simulink model "frameBasedSobelFilter"  (R2023a)
settings: Solver=FixedStepDiscrete  StartTime=0.0  StopTime=2  RelTol=1e-3
values from neighbouring files (symbols this model uses):
  c = 752    [setupFrame.m]
  r = 480    [setupFrame.m]
libraries: hdlsllib x16, visionsources x1
Description:
  | Sobel Edge Detection Using the MATLAB(R) Function Block
  | This example shows how to use HDL Coder(TM) to check,
  | generate, and verify HDL code for a Sobel Edge Detection
  | block built using the MATLAB Function block.
settings Model: Creator=The MathWorks, Inc.  LastModifiedBy=dskap
settings SolverCC: AlgebraicLoopSolver=TrustRegion
settings DataIOCC: LimitDataPoints=on  SaveFormat=Array  SignalLogging=off  ReturnWorkspaceOutputs=off
settings OptimizationCC: BlockReduction=off  ConditionallyExecuteInputs=off  DefaultParameterBehavior=Inlined  ExpressionDepthLimit=2147483647  InitFltsAndDblsToZero=on  EfficientMapNaN2IntZero=off  LifeSpan=inf
settings DebuggingCC: AlgebraicLoopMsg=error  SaveWithParameterizedLinksMsg=none  UnderspecifiedInitializationDetection=Classic  MergeDetectMultiDrivingBlocksExec=none  SignalResolutionControl=TryResolveAllWithWarning  MultiTaskDSMMsg=warning  MultiTaskCondExecSysMsg=none  SingleTaskRateTransMsg=error  IntegerOverflowMsg=none  ParameterPrecisionLossMsg=none  FcnCallInpInsideContextMsg=warning  UnconnectedInputMsg=warning  UnconnectedOutputMsg=warning  UnconnectedLineMsg=warning  AllowSymbolicDim=off  StateNameClashWarn=warning  StrictBusMsg=ErrorOnBusTreatedAsVector  SFUnexpectedBacktrackingDiag=warning  SFNoUnconditionalDefaultTransitionDiag=warning  SFExecutionAtInitializationDiag=none  IntegerSaturationMsg=none  ArithmeticOperatorsInVariantConditions=warning
settings HardwareCC: ProdBitPerPointer=32  ProdBitPerSizeT=32  ProdBitPerPtrDiffT=32  ProdLargestAtomicFloat=None  ProdIntDivRoundTo=Undefined  ProdEndianess=Unspecified  ProdWordSize=32  ProdHWDeviceType=ASIC/FPGA  TargetHWDeviceType=32-bit Generic  ProdEqTarget=off
settings ModelReferenceCC: EnableRefExpFcnMdlSchedulingChecks=on  PropagateSignalLabelsOutOfModel=off
settings SFSimCC: SimUseLocalCustomCode=off  CustomCodeUndefinedFunction=UseInterfaceOnly
settings RTWCC: RTWUseLocalCustomCode=off  DLArmComputeVersion=19.05
settings CodeAppCC: StateflowObjectComments=on
settings GRTTargetCC: TargetFcnLib=ansi_tfl_tmw.mat  TargetLangStandard=C89/C90 (ANSI)  CombineOutputUpdateFcns=off  GRTInterface=on
settings ConfigComp: CovMetricSettings=dw  CovSaveCumulativeToWorkspaceVar=on  CovSaveSingleToWorkspaceVar=on  CovExternalEMLEnable=off

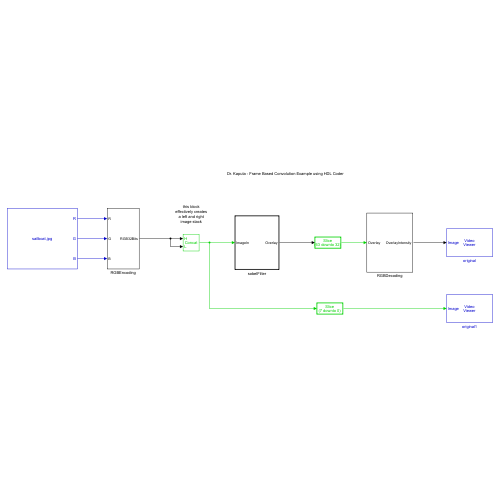
[thumbnail: Simulink's stored preview of the top-level diagram]
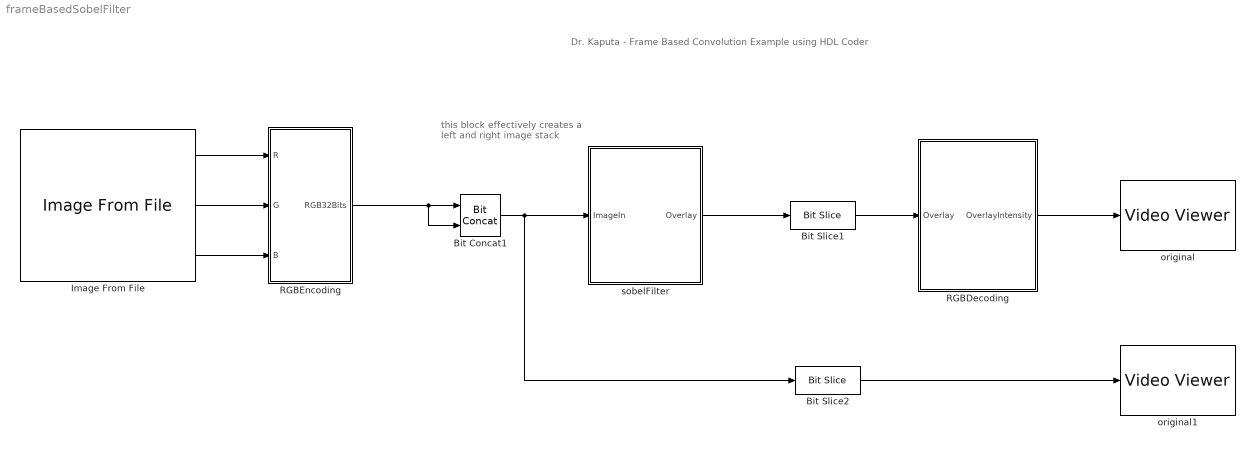
== system frameBasedSobelFilter ==
  note: this block effectively creates a left and right image stack
  note: Dr. Kaputa - Frame Based Convolution Example using HDL Coder
  Bit Concat1 : hdlsllib/Logic and Bit Operations/Bit Concat  numInputs=2
  Bit Slice1 : hdlsllib/Logic and Bit Operations/Bit Slice  lidx=63  ridx=32
  Bit Slice2 : hdlsllib/Logic and Bit Operations/Bit Slice  lidx=7  ridx=0
  Image From File : visionsources/Image From File  Tag=vipblks_nd  FileName=sailboat.jpg  Ts=1  imagePorts=Separate color signals  OutPortLabels=R|G|B  ImageDataType=Inherit from input image  sdImageDataType=uint(8)  Signed=on  WordLength=16  FractionLengthMode=User-defined  FractionLength=15
  RGBDecoding : Subsystem
  RGBEncoding : Subsystem
  original : VideoViewer  FigPos=[-1279 718 1280 622.666666666667]
  original1 : VideoViewer  FigPos=[-1279 718 1280 622.666666666667]
  sobelFilter : Subsystem  TreatAsAtomicUnit=on
  wires:
  sobelFilter/1(Overlay) -> Bit Slice1/1
  Image From File/1 -> RGBEncoding/1(R)
  Image From File/2 -> RGBEncoding/2(G)
  Image From File/3 -> RGBEncoding/3(B)
  RGBEncoding/1(RGB32Bits) -> Bit Concat1/2, Bit Concat1/1
  Bit Concat1/1 -> Bit Slice2/1, sobelFilter/1(ImageIn)
  RGBDecoding/1(OverlayIntensity) -> original/1
  Bit Slice1/1 -> RGBDecoding/1(Overlay)
  Bit Slice2/1 -> original1/1

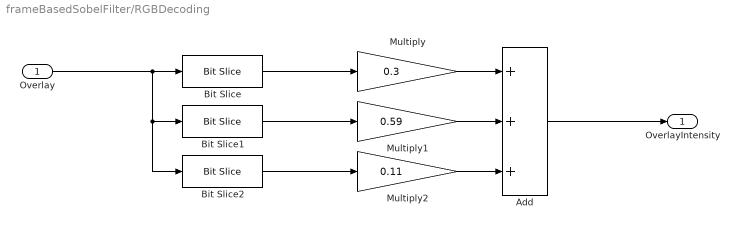
== system frameBasedSobelFilter/RGBDecoding ==
  Overlay : Inport
  Add : Sum  Inputs=+++  OutDataTypeStr=uint8
  Bit Slice : hdlsllib/Logic and Bit Operations/Bit Slice  lidx=23  ridx=16
  Bit Slice1 : hdlsllib/Logic and Bit Operations/Bit Slice  lidx=15  ridx=8
  Bit Slice2 : hdlsllib/Logic and Bit Operations/Bit Slice  lidx=7  ridx=0
  Multiply : Gain  Gain=0.3  OutDataTypeStr=uint8
  Multiply1 : Gain  Gain=0.59  OutDataTypeStr=uint8
  Multiply2 : Gain  Gain=0.11  OutDataTypeStr=uint8
  OverlayIntensity : Outport
  wires:
  Multiply/1 -> Add/1
  Overlay/1 -> Bit Slice2/1, Bit Slice1/1, Bit Slice/1
  Bit Slice/1 -> Multiply/1
  Bit Slice2/1 -> Multiply2/1
  Add/1 -> OverlayIntensity/1
  Bit Slice1/1 -> Multiply1/1
  Multiply2/1 -> Add/3
  Multiply1/1 -> Add/2

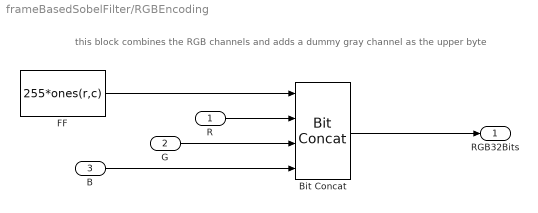
== system frameBasedSobelFilter/RGBEncoding ==
  note: this block combines the RGB channels and adds a dummy gray channel as the upper byte
  R : Inport
  G : Inport  Port=2
  B : Inport  Port=3
  Bit Concat : hdlsllib/Logic and Bit Operations/Bit Concat  numInputs=4
  FF : Constant  Value=255*ones(r,c)  OutDataTypeStr=uint8  SampleTime=1
  RGB32Bits : Outport
  wires:
  FF/1 -> Bit Concat/1
  Bit Concat/1 -> RGB32Bits/1
  R/1 -> Bit Concat/2
  G/1 -> Bit Concat/3
  B/1 -> Bit Concat/4

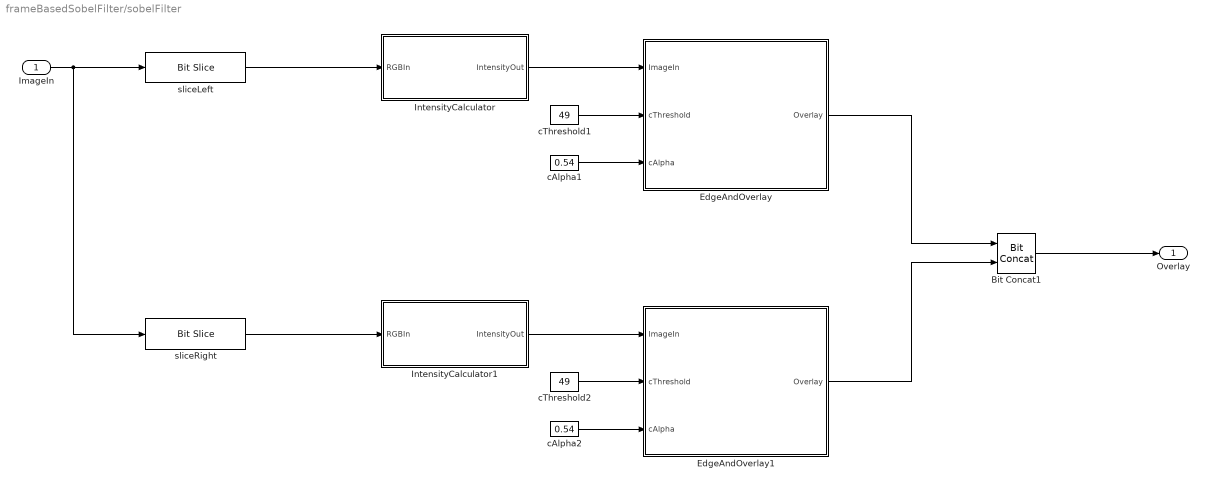
== system frameBasedSobelFilter/sobelFilter ==
  ImageIn : Inport
  Bit Concat1 : hdlsllib/Logic and Bit Operations/Bit Concat  numInputs=2
  EdgeAndOverlay : MATLAB Function  TreatAsAtomicUnit=on
  EdgeAndOverlay1 : MATLAB Function  TreatAsAtomicUnit=on
  IntensityCalculator : Subsystem
  IntensityCalculator1 : Subsystem
  cAlpha1 : Constant  Value=0.54  OutDataTypeStr=fixdt(0,16,15)  SampleTime=1
  cAlpha2 : Constant  Value=0.54  OutDataTypeStr=fixdt(0,16,15)  SampleTime=1
  cThreshold1 : Constant  Value=49  OutDataTypeStr=uint8  SampleTime=1
  cThreshold2 : Constant  Value=49  OutDataTypeStr=uint8  SampleTime=1
  sliceLeft : hdlsllib/Logic and Bit Operations/Bit Slice  lidx=63  ridx=32
  sliceRight : hdlsllib/Logic and Bit Operations/Bit Slice  lidx=31  ridx=0
  Overlay : Outport
  wires:
  cThreshold1/1 -> EdgeAndOverlay/2(cThreshold)
  cAlpha1/1 -> EdgeAndOverlay/3(cAlpha)
  IntensityCalculator/1(IntensityOut) -> EdgeAndOverlay/1(ImageIn)
  sliceLeft/1 -> IntensityCalculator/1(RGBIn)
  ImageIn/1 -> sliceLeft/1, sliceRight/1
  sliceRight/1 -> IntensityCalculator1/1(RGBIn)
  IntensityCalculator1/1(IntensityOut) -> EdgeAndOverlay1/1(ImageIn)
  cAlpha2/1 -> EdgeAndOverlay1/3(cAlpha)
  EdgeAndOverlay1/1(Overlay) -> Bit Concat1/2
  cThreshold2/1 -> EdgeAndOverlay1/2(cThreshold)
  Bit Concat1/1 -> Overlay/1
  EdgeAndOverlay/1(Overlay) -> Bit Concat1/1

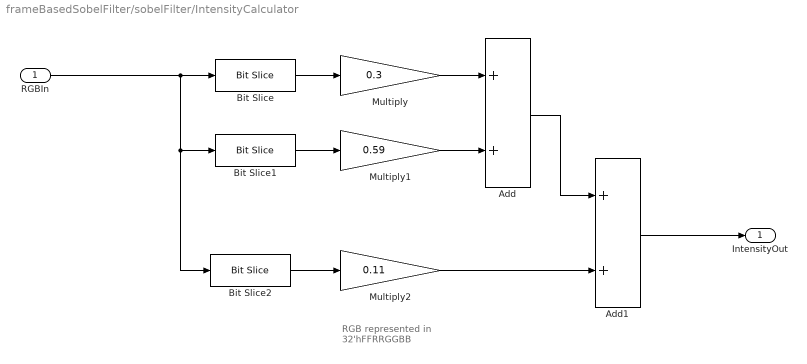
== system frameBasedSobelFilter/sobelFilter/IntensityCalculator ==
  note: RGB represented in
      | 32'hFFRRGGBB
  RGBIn : Inport
  Add : Sum  OutDataTypeStr=uint8
  Add1 : Sum  OutDataTypeStr=uint8
  Bit Slice : hdlsllib/Logic and Bit Operations/Bit Slice  lidx=23  ridx=16
  Bit Slice1 : hdlsllib/Logic and Bit Operations/Bit Slice  lidx=15  ridx=8
  Bit Slice2 : hdlsllib/Logic and Bit Operations/Bit Slice  lidx=7  ridx=0
  Multiply : Gain  Gain=0.3  OutDataTypeStr=uint8
  Multiply1 : Gain  Gain=0.59  OutDataTypeStr=uint8
  Multiply2 : Gain  Gain=0.11  OutDataTypeStr=uint8
  IntensityOut : Outport
  wires:
  Bit Slice1/1 -> Multiply1/1
  Multiply2/1 -> Add1/2
  Multiply/1 -> Add/1
  Multiply1/1 -> Add/2
  Bit Slice/1 -> Multiply/1
  Add/1 -> Add1/1
  RGBIn/1 -> Bit Slice2/1, Bit Slice1/1, Bit Slice/1
  Add1/1 -> IntensityOut/1
  Bit Slice2/1 -> Multiply2/1

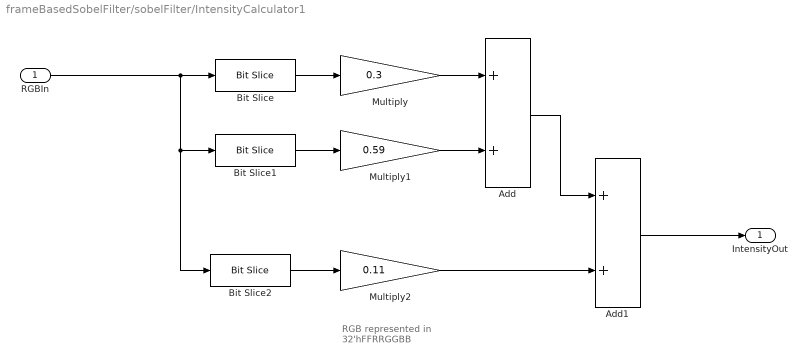
== system frameBasedSobelFilter/sobelFilter/IntensityCalculator1 ==
  note: RGB represented in
      | 32'hFFRRGGBB
  RGBIn : Inport
  Add : Sum  OutDataTypeStr=uint8
  Add1 : Sum  OutDataTypeStr=uint8
  Bit Slice : hdlsllib/Logic and Bit Operations/Bit Slice  lidx=23  ridx=16
  Bit Slice1 : hdlsllib/Logic and Bit Operations/Bit Slice  lidx=15  ridx=8
  Bit Slice2 : hdlsllib/Logic and Bit Operations/Bit Slice  lidx=7  ridx=0
  Multiply : Gain  Gain=0.3  OutDataTypeStr=uint8
  Multiply1 : Gain  Gain=0.59  OutDataTypeStr=uint8
  Multiply2 : Gain  Gain=0.11  OutDataTypeStr=uint8
  IntensityOut : Outport
  wires:
  Bit Slice1/1 -> Multiply1/1
  Multiply2/1 -> Add1/2
  Multiply/1 -> Add/1
  Multiply1/1 -> Add/2
  Bit Slice/1 -> Multiply/1
  Add/1 -> Add1/1
  RGBIn/1 -> Bit Slice2/1, Bit Slice1/1, Bit Slice/1
  Add1/1 -> IntensityOut/1
  Bit Slice2/1 -> Multiply2/1

== matlab function frameBasedSobelFilter/sobelFilter/EdgeAndOverlay1 ==
  data: Overlay output; ImageIn input; cThreshold input; cAlpha input
function Overlay   = edgeDetectionAndOverlay(ImageIn, cThreshold, cAlpha)
 
E = hdl.npufun(@sobel_kernel, [3 3], ImageIn, 'NonSampleInput', cThreshold);
Overlay = hdl.npufun(@mix_kernel, [1 1], E, ImageIn, 'NonSampleInput', cAlpha);
 
end
 
function e = sobel_kernel(in, cThreshold)
 
u = fi(in);
% products
hp1delay = coder.hdl.pipeline(u(1),1);
hp2 = fi(2)*u(2);
hp2delay = coder.hdl.pipeline(hp2,1);
ha1 = hp1delay + hp2delay;
ha1delay = coder.hdl.pipeline(ha1,1);
u3delay = coder.hdl.pipeline(u(3),2);
ha2 = ha1delay + u3delay;
ha2delay = coder.hdl.pipeline(ha2,1);
 
hp11delay = coder.hdl.pipeline(u(7),1);
hp22 = fi(2)*u(8);
hp22delay = coder.hdl.pipeline(hp22,1);
ha11 = hp11delay + hp22delay;
ha11delay = coder.hdl.pipeline(ha11,1);
u9delay = coder.hdl.pipeline(u(9),2);
ha22 = ha11delay + u9delay;
ha22delay = coder.hdl.pipeline(ha22,1);
 
hGrad = ha2delay - ha22delay;
 
vp1delay = coder.hdl.pipeline(u(1),1);
vp2 = fi(2)*u(4);
vp2delay = coder.hdl.pipeline(vp2,1);
va1 = vp1delay + vp2delay;
va1delay = coder.hdl.pipeline(va1,1);
u7delay = coder.hdl.pipeline(u(7),2);
va2 = va1delay + u7delay;
va2delay = coder.hdl.pipeline(va2,1);
 
vp11delay = coder.hdl.pipeline(u(3),1);
vp22 = fi(2)*u(6);
vp22delay = coder.hdl.pipeline(vp22,1);
va11 = vp11delay + vp22delay;
va11delay = coder.hdl.pipeline(va11,1);
u9delay = coder.hdl.pipeline(u(9),2);
va22 = va11delay + u9delay;
va22delay = coder.hdl.pipeline(va22,1);
 
vGrad = va2delay - va22delay;
 
hGrad1 = bitshift(hGrad, -3); % Divide by 8
vGrad1 = bitshift(vGrad, -3); % Divide by 8
 
hGrad = coder.hdl.pipeline(hGrad1,2);
vGrad = coder.hdl.pipeline(vGrad1,2);
hprod1 = hGrad*hGrad;
vprod1 = vGrad*vGrad;
hprodDelay = coder.hdl.pipeline(hprod1,4);
vprodDelay = coder.hdl.pipeline(vprod1,4);
thresholdValueSq = fi(cThreshold); % Threshold parameter
ad1 = (hprodDelay + vprodDelay);
ad1Delay = coder.hdl.pipeline(ad1,1);
ed = ad1Delay > thresholdValueSq;
e = coder.hdl.pipeline(ed,2);

end
 
function O = mix_kernel(E, I, cAlpha)
 
alpha = fi(cAlpha); % Parameter for combining images
scaleE = E*fi(255,0,8,0);
scaleEdelay = coder.hdl.pipeline(scaleE,2);
O1 = scaleEdelay*(1-alpha);
O1delay = coder.hdl.pipeline(O1,2);
O2 = I*alpha;
O2delay = coder.hdl.pipeline(O2,4);
val = O1delay + O2delay;
val = fi(val,0,8,0);
O = bitconcat(fi(255,0,8,0),val,val,val); 
end

== matlab function frameBasedSobelFilter/sobelFilter/EdgeAndOverlay ==
  data: Overlay output; ImageIn input; cThreshold input; cAlpha input
function Overlay   = edgeDetectionAndOverlay(ImageIn, cThreshold, cAlpha)
 
E = hdl.npufun(@sobel_kernel, [3 3], ImageIn, 'NonSampleInput', cThreshold);
Overlay = hdl.npufun(@mix_kernel, [1 1], E, ImageIn, 'NonSampleInput', cAlpha);
 
end
 
function e = sobel_kernel(in, cThreshold)
 
u = fi(in);
% products
hp1delay = coder.hdl.pipeline(u(1),1);
hp2 = fi(2)*u(2);
hp2delay = coder.hdl.pipeline(hp2,1);
ha1 = hp1delay + hp2delay;
ha1delay = coder.hdl.pipeline(ha1,1);
u3delay = coder.hdl.pipeline(u(3),2);
ha2 = ha1delay + u3delay;
ha2delay = coder.hdl.pipeline(ha2,1);
 
hp11delay = coder.hdl.pipeline(u(7),1);
hp22 = fi(2)*u(8);
hp22delay = coder.hdl.pipeline(hp22,1);
ha11 = hp11delay + hp22delay;
ha11delay = coder.hdl.pipeline(ha11,1);
u9delay = coder.hdl.pipeline(u(9),2);
ha22 = ha11delay + u9delay;
ha22delay = coder.hdl.pipeline(ha22,1);
 
hGrad = ha2delay - ha22delay;
 
vp1delay = coder.hdl.pipeline(u(1),1);
vp2 = fi(2)*u(4);
vp2delay = coder.hdl.pipeline(vp2,1);
va1 = vp1delay + vp2delay;
va1delay = coder.hdl.pipeline(va1,1);
u7delay = coder.hdl.pipeline(u(7),2);
va2 = va1delay + u7delay;
va2delay = coder.hdl.pipeline(va2,1);
 
vp11delay = coder.hdl.pipeline(u(3),1);
vp22 = fi(2)*u(6);
vp22delay = coder.hdl.pipeline(vp22,1);
va11 = vp11delay + vp22delay;
va11delay = coder.hdl.pipeline(va11,1);
u9delay = coder.hdl.pipeline(u(9),2);
va22 = va11delay + u9delay;
va22delay = coder.hdl.pipeline(va22,1);
 
vGrad = va2delay - va22delay;
 
hGrad1 = bitshift(hGrad, -3); % Divide by 8
vGrad1 = bitshift(vGrad, -3); % Divide by 8
 
hGrad = coder.hdl.pipeline(hGrad1,2);
vGrad = coder.hdl.pipeline(vGrad1,2);
hprod1 = hGrad*hGrad;
vprod1 = vGrad*vGrad;
hprodDelay = coder.hdl.pipeline(hprod1,4);
vprodDelay = coder.hdl.pipeline(vprod1,4);
thresholdValueSq = fi(cThreshold); % Threshold parameter
ad1 = (hprodDelay + vprodDelay);
ad1Delay = coder.hdl.pipeline(ad1,1);
ed = ad1Delay > thresholdValueSq;
e = coder.hdl.pipeline(ed,2);

end
 
function O = mix_kernel(E, I, cAlpha)
 
alpha = fi(cAlpha); % Parameter for combining images
scaleE = E*fi(255,0,8,0);
scaleEdelay = coder.hdl.pipeline(scaleE,2);
O1 = scaleEdelay*(1-alpha);
O1delay = coder.hdl.pipeline(O1,2);
O2 = I*alpha;
O2delay = coder.hdl.pipeline(O2,4);
val = O1delay + O2delay;
val = fi(val,0,8,0);
O = bitconcat(fi(255,0,8,0),val,val,val); 
end
